simulink library "lib_Labor_PMA"  (R2020a)
settings: Solver=VariableStepAuto  StartTime=0.0  StopTime=10.0  RelTol=1e-3
settings Model: Creator=manuel  LastModifiedBy=student_prsr
settings OptimizationCC: ZeroExternalMemoryAtStartup=off  ZeroInternalMemoryAtStartup=off
settings SFSimCC: SimUseLocalCustomCode=off  SimParseCustomCode=off
settings RTWCC: RTWUseLocalCustomCode=off  TargetLang=C++
settings GRTTargetCC: TargetLangStandard=C++03 (ISO)  MultiInstanceERTCode=on  CodeInterfacePackaging=C++ class

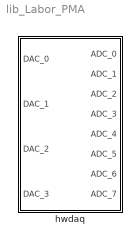
== system lib_Labor_PMA ==
  hwdaq : Subsystem  mask(SPI_write_read){}
      mask help:
      | Write to to DAC via SPI.
      | Read from ADC via SPI:

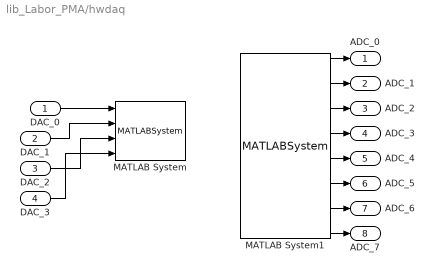
== system lib_Labor_PMA/hwdaq ==
  DAC_0 : Inport
  DAC_1 : Inport  Port=2
  DAC_2 : Inport  Port=3
  DAC_3 : Inport  Port=4
  MATLAB System : MATLABSystem  System=hwdac  SimulateUsing=Code generation
      mask Type: hwdac
      mask Display:
      | disp('hwdac');
      | port_label('input',1,'DAC_0');
      | port_label('input',2,'DAC_1');
      | port_label('input',3,'DAC_2');
      | port_label('input',4,'DAC_3');
  MATLAB System1 : MATLABSystem  System=hwadc  SimulateUsing=Code generation
      mask Type: hwadc
      mask Display:
      | disp('hwadc');
      | port_label('output',1,'adcValues0');
      | port_label('output',2,'adcValues1');
      | port_label('output',3,'adcValues2');
      | port_label('output',4,'adcValues3');
      | port_label('output',5,'adcValues4');
      | port_label('output',6,'adcValues5');
      | port_label('output',7,'adcValues6');
      | port_label('output',8,'adcValues7');
  ADC_0 : Outport
  ADC_1 : Outport  Port=2
  ADC_2 : Outport  Port=3
  ADC_3 : Outport  Port=4
  ADC_4 : Outport  Port=5
  ADC_5 : Outport  Port=6
  ADC_6 : Outport  Port=7
  ADC_7 : Outport  Port=8
  wires:
  MATLAB System1/7 -> ADC_6/1
  MATLAB System1/1 -> ADC_0/1
  MATLAB System1/4 -> ADC_3/1
  MATLAB System1/2 -> ADC_1/1
  MATLAB System1/6 -> ADC_5/1
  MATLAB System1/5 -> ADC_4/1
  MATLAB System1/3 -> ADC_2/1
  MATLAB System1/8 -> ADC_7/1
  DAC_0/1 -> MATLAB System/1
  DAC_1/1 -> MATLAB System/2
  DAC_2/1 -> MATLAB System/3
  DAC_3/1 -> MATLAB System/4
